simulink model "EngBrk_VNTP"  (R2016b)
settings: configuration reference "CodeGenConfigSet" (kept outside this file)
values from neighbouring files (symbols this model uses):
  COETS_EBSTATE_BRAKED = uint16(1)    [init_EngBrk_VNTP.m]
  ENGBRK_FIRED = uint8(0)    [init_EngBrk_VNTP.m]
  EngBrk_nEISGovOff_C = Calibration.Parameter    [init_EngBrk_VNTP.m]
  EngBrk_nEng_CUR = Calibration.Parameter    [init_EngBrk_VNTP.m]
  EngBrk_nEng_CURX = Calibration.Parameter    [init_EngBrk_VNTP.m]
  EngBrk_nEngThres_C = Calibration.Parameter    [init_EngBrk_VNTP.m]
  EngBrk_nOfsCA_CUR = Calibration.Parameter    [init_EngBrk_VNTP.m]
  EngBrk_nOfsCA_CURX = Calibration.Parameter    [init_EngBrk_VNTP.m]
  EngBrk_nOfsCADfct_C = Calibration.Parameter    [init_EngBrk_VNTP.m]
  EngBrk_rECRVlv_CUR = Calibration.Parameter    [init_EngBrk_VNTP.m]
  EngBrk_rECRVlv_CURX = Calibration.Parameter    [init_EngBrk_VNTP.m]
  EngBrk_rECRVlvHighDev_C = Calibration.Parameter    [init_EngBrk_VNTP.m]
  EngBrk_rECRVlvLowDev_C = Calibration.Parameter    [init_EngBrk_VNTP.m]
  EngBrk_rExhFlp_CUR = Calibration.Parameter    [init_EngBrk_VNTP.m]
  EngBrk_rExhFlp_CURX = Calibration.Parameter    [init_EngBrk_VNTP.m]
  EngBrk_rExhFlpHighDev_C = Calibration.Parameter    [init_EngBrk_VNTP.m]
  EngBrk_rExhFlpLowDev_C = Calibration.Parameter    [init_EngBrk_VNTP.m]
  EngBrk_rPT1TrqCurr_C = Calibration.Parameter    [init_EngBrk_VNTP.m]
  EngBrk_stDemMsk_C = Calibration.Parameter    [init_EngBrk_VNTP.m]
  EngBrk_swtECRVlv_C = Calibration.Parameter    [init_EngBrk_VNTP.m]
  EngBrk_swtExhFlp_C = Calibration.Parameter    [init_EngBrk_VNTP.m]
  EngBrk_tiDelayExhOff_C = Calibration.Parameter    [init_EngBrk_VNTP.m]
  EngBrk_tiPT1TrqCurr_C = Calibration.Parameter    [init_EngBrk_VNTP.m]
  EngBrk_tiRmp_C = Calibration.Parameter    [init_EngBrk_VNTP.m]
  EngBrk_tiRmpBlowOff_C = Calibration.Parameter    [init_EngBrk_VNTP.m]
  EngBrk_trqDeltaEnabECRVlv_GCUR = Calibration.Parameter    [init_EngBrk_VNTP.m]
  EngBrk_trqDeltaEnabECRVlv_GCURX = Calibration.Parameter    [init_EngBrk_VNTP.m]
  EngBrk_trqDeltaEnabExh_GCUR = Calibration.Parameter    [init_EngBrk_VNTP.m]
  EngBrk_trqDeltaEnabExh_GCURX = Calibration.Parameter    [init_EngBrk_VNTP.m]
  EngBrk_trqLimEnabECRVlv_GCUR = Calibration.Parameter    [init_EngBrk_VNTP.m]
  EngBrk_trqLimEnabECRVlv_GCURX = Calibration.Parameter    [init_EngBrk_VNTP.m]
  EngBrk_trqLimEnabExh_GCUR = Calibration.Parameter    [init_EngBrk_VNTP.m]
  EngBrk_trqLimEnabExh_GCURX = Calibration.Parameter    [init_EngBrk_VNTP.m]
  EngBrk_trqMax_GCUR = Calibration.Parameter    [init_EngBrk_VNTP.m]
  EngBrk_trqMax_GCURX = Calibration.Parameter    [init_EngBrk_VNTP.m]
  EngBrk_trqMaxDfct1_GCUR = Calibration.Parameter    [init_EngBrk_VNTP.m]
  EngBrk_trqMaxDfct1_GCURX = Calibration.Parameter    [init_EngBrk_VNTP.m]
  EngBrk_trqMaxDfct2_GCUR = Calibration.Parameter    [init_EngBrk_VNTP.m]
  EngBrk_trqMaxDfct2_GCURX = Calibration.Parameter    [init_EngBrk_VNTP.m]
  EngBrk_trqMaxDfct3_GCUR = Calibration.Parameter    [init_EngBrk_VNTP.m]
  EngBrk_trqMaxDfct3_GCURX = Calibration.Parameter    [init_EngBrk_VNTP.m]
  PRC_100 = uint8(0)    [init_EngBrk_VNTP.m]
  TRQ_MIN = int16(-3276)    [init_EngBrk_VNTP.m]
undefined symbols (not defined in the file or in its folder): EngBrk_VNTP_DT, HPUn_etaPmp_MAPY, Switch_conv
libraries: simulink x17, CXLib x10
settings Model: Creator=lenovo  LastModifiedBy=wangrui
settings ConfigSetRef: SourceLocation=Base Workspace

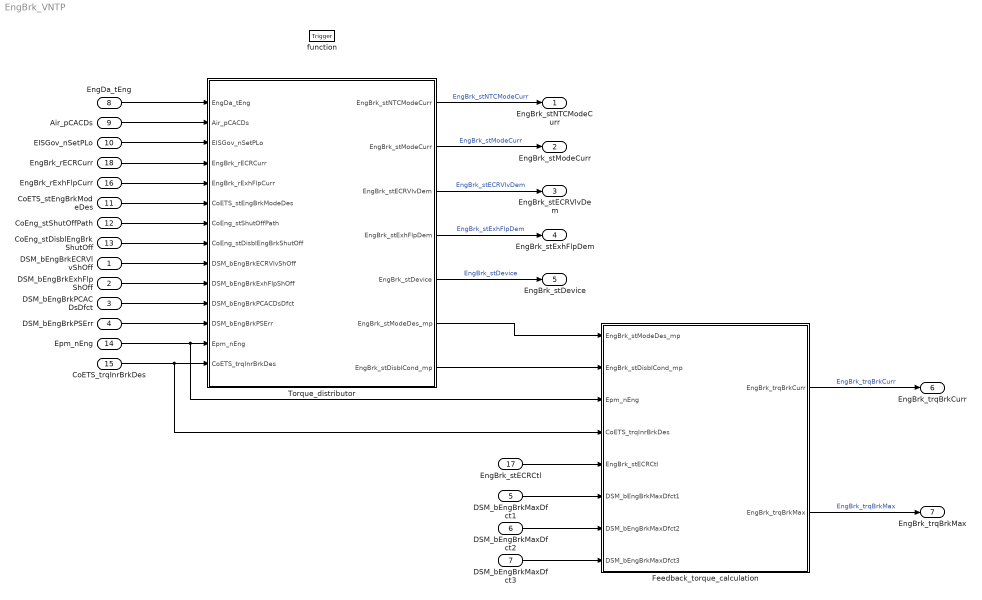
== system EngBrk_VNTP ==
  DSM_bEngBrkECRVlvShOff : Inport  Description=state of FId_EngBrkECRVlvShOff  OutMin=0  OutMax=1  OutDataTypeStr=boolean
  DSM_bEngBrkExhFlpShOff : Inport  Description=state of FId_EngBrkExhFlpShOff  Port=2  OutMin=0  OutMax=1  OutDataTypeStr=boolean
  DSM_bEngBrkPCACDsDfct : Inport  Description=state of FId_EngBrkPCACDsDfct  Port=3  OutMin=0  OutMax=1  OutDataTypeStr=boolean
  DSM_bEngBrkPSErr : Inport  Description=state of FId_EngBrkPSErr  Port=4  OutMin=0  OutMax=1  OutDataTypeStr=boolean
  DSM_bEngBrkMaxDfct1 : Inport  Description=state of FId_EngBrkMaxDfct1  Port=5  OutMin=0  OutMax=1  OutDataTypeStr=boolean
  DSM_bEngBrkMaxDfct2 : Inport  Description=state of FId_EngBrkMaxDfct2  Port=6  OutMin=0  OutMax=1  OutDataTypeStr=boolean
  DSM_bEngBrkMaxDfct3 : Inport  Description=state of FId_EngBrkMaxDfct3  Port=7  OutMin=0  OutMax=1  OutDataTypeStr=boolean
  EngDa_tEng : Inport  Tag=deg  Description=Engine temperature  Port=8  OutMin=-1000  OutMax=1000  OutDataTypeStr=Temp_deg
  Air_pCACDs : Inport  Tag=kPa  Description=Air pressure downstream of the charge air cooler  Port=9  OutMin=-3276.8  OutMax=3276.7  OutDataTypeStr=AirPressure_kPa
  EISGov_nSetPLo : Inport  Tag=rpm  Description=Lower limit of the speed interval (set point speed) of the EISGov  Port=10  OutMin=-12000  OutMax=12000  OutDataTypeStr=EngSpeed_rpm
  CoETS_stEngBrkModeDes : Inport  Description=Desired mode to VNTP  Port=11  OutMin=0  OutMax=65535  OutDataTypeStr=State_uint16
  CoEng_stShutOffPath : Inport  Description=Active shut-off paths resulting from active reversible,irreversible and afterrun shut-off paths  Port=12  OutMin=0  OutMax=65535  OutDataTypeStr=State_uint16
  CoEng_stDisblEngBrkShutOff : Inport  Description=|  Port=13  OutMin=0  OutMax=1  OutDataTypeStr=boolean
      | Status if injections are enabled although engine
      | brake can be active
  Epm_nEng : Inport  Tag=rpm  Description=Engine speed  Port=14  OutMin=0  OutMax=6000  OutDataTypeStr=EngSpeed_rpm
  CoETS_trqInrBrkDes : Inport  Tag=Nm  Description=Desired torque to VNTP Nm  Port=15  OutMin=-3276.8  OutMax=3276.7  OutDataTypeStr=Trq_Nm
  EngBrk_rExhFlpCurr : Inport  Tag=%  Description=Actual status (process signal) of exhaust flap  Port=16  OutMin=-200  OutMax=200  OutDataTypeStr=DutyCycle_rate
  EngBrk_stECRCtl : Inport  Description=Current status of the Engine compression release Valve(ECRVlv)  Port=17  OutMin=0  OutMax=255  OutDataTypeStr=State_uint8
  EngBrk_rECRCurr : Inport  Tag=%  Description=Current status of the Engine compression release Valve(ECRVlv) state machine  Port=18  OutMin=-200  OutMax=200  OutDataTypeStr=DutyCycle_rate
  function : TriggerPort  TriggerType=function-call  VariantControl=Variant
  Feedback_torque_calculation : Subsystem
  Torque_distributor : Subsystem
  EngBrk_stNTCModeCurr : Outport  Description=VNTP status for NTC, TRUE if active (CRER or ExhFlp)  OutMin=0  OutMax=255  OutDataTypeStr=State_uint8
  EngBrk_stModeCurr : Outport  Description=VNTP status, TRUE if active (CRER or ExhFlp and injection shut-off)  Port=2  OutMin=0  OutMax=255  OutDataTypeStr=State_uint8
  EngBrk_stECRVlvDem : Outport  Description=Activation demand to Engine compression release Valve(ECRVlv)  Port=3  OutMin=0  OutMax=255  OutDataTypeStr=State_uint8
  EngBrk_stExhFlpDem : Outport  Description=Activation demand to exhaust flap  Port=4  OutMin=0  OutMax=1  OutDataTypeStr=boolean
  EngBrk_stDevice : Outport  Description=Device actuated by VNTP, used as map selection for ratio and pressure setpoint calculation  Port=5  OutMin=0  OutMax=255  OutDataTypeStr=State_uint8
  EngBrk_trqBrkCurr : Outport  Tag=Nm  Description=Current engine brake torque  Port=6  OutMin=-3276.8  OutMax=3276.7  OutDataTypeStr=Trq_Nm
  EngBrk_trqBrkMax : Outport  Tag=Nm  Description=Maximum available engine brake torque  Port=7  OutMin=-3276.8  OutMax=3276.7  OutDataTypeStr=Trq_Nm
  wires:
  EngBrk_rECRCurr/1 -> Torque_distributor/4(EngBrk_rECRCurr)
  Epm_nEng/1 -> Feedback_torque_calculation/3(Epm_nEng), Torque_distributor/13(Epm_nEng)
  Torque_distributor/4(EngBrk_stExhFlpDem) -> EngBrk_stExhFlpDem/1  "EngBrk_stExhFlpDem"
  EISGov_nSetPLo/1 -> Torque_distributor/3(EISGov_nSetPLo)
  CoETS_trqInrBrkDes/1 -> Feedback_torque_calculation/4(CoETS_trqInrBrkDes), Torque_distributor/14(CoETS_trqInrBrkDes)
  CoEng_stDisblEngBrkShutOff/1 -> Torque_distributor/8(CoEng_stDisblEngBrkShutOff)
  Air_pCACDs/1 -> Torque_distributor/2(Air_pCACDs)
  Torque_distributor/2(EngBrk_stModeCurr) -> EngBrk_stModeCurr/1  "EngBrk_stModeCurr"
  Torque_distributor/7(EngBrk_stDisblCond_mp) -> Feedback_torque_calculation/2(EngBrk_stDisblCond_mp)
  Torque_distributor/3(EngBrk_stECRVlvDem) -> EngBrk_stECRVlvDem/1  "EngBrk_stECRVlvDem"
  Feedback_torque_calculation/2(EngBrk_trqBrkMax) -> EngBrk_trqBrkMax/1  "EngBrk_trqBrkMax"
  Feedback_torque_calculation/1(EngBrk_trqBrkCurr) -> EngBrk_trqBrkCurr/1  "EngBrk_trqBrkCurr"
  Torque_distributor/5(EngBrk_stDevice) -> EngBrk_stDevice/1  "EngBrk_stDevice"
  CoETS_stEngBrkModeDes/1 -> Torque_distributor/6(CoETS_stEngBrkModeDes)
  EngBrk_stECRCtl/1 -> Feedback_torque_calculation/5(EngBrk_stECRCtl)
  CoEng_stShutOffPath/1 -> Torque_distributor/7(CoEng_stShutOffPath)
  Torque_distributor/6(EngBrk_stModeDes_mp) -> Feedback_torque_calculation/1(EngBrk_stModeDes_mp)
  EngDa_tEng/1 -> Torque_distributor/1(EngDa_tEng)
  EngBrk_rExhFlpCurr/1 -> Torque_distributor/5(EngBrk_rExhFlpCurr)
  Torque_distributor/1(EngBrk_stNTCModeCurr) -> EngBrk_stNTCModeCurr/1  "EngBrk_stNTCModeCurr"
  DSM_bEngBrkMaxDfct1/1 -> Feedback_torque_calculation/6(DSM_bEngBrkMaxDfct1)
  DSM_bEngBrkMaxDfct2/1 -> Feedback_torque_calculation/7(DSM_bEngBrkMaxDfct2)
  DSM_bEngBrkMaxDfct3/1 -> Feedback_torque_calculation/8(DSM_bEngBrkMaxDfct3)
  DSM_bEngBrkECRVlvShOff/1 -> Torque_distributor/9(DSM_bEngBrkECRVlvShOff)
  DSM_bEngBrkExhFlpShOff/1 -> Torque_distributor/10(DSM_bEngBrkExhFlpShOff)
  DSM_bEngBrkPCACDsDfct/1 -> Torque_distributor/11(DSM_bEngBrkPCACDsDfct)
  DSM_bEngBrkPSErr/1 -> Torque_distributor/12(DSM_bEngBrkPSErr)

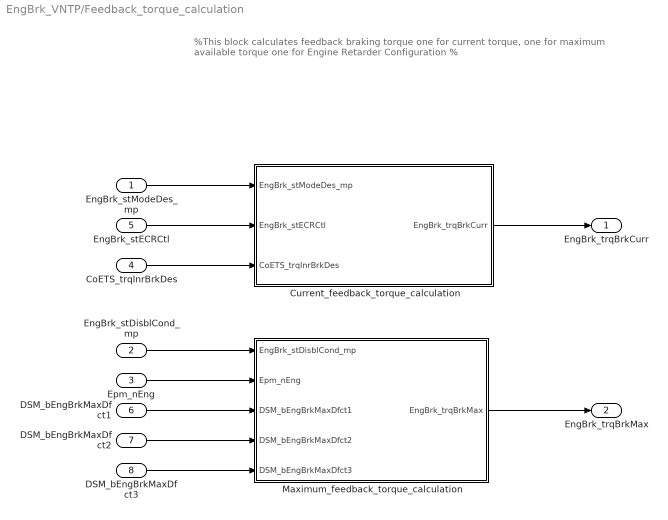
== system EngBrk_VNTP/Feedback_torque_calculation ==
  note: %This block calculates feedback braking torque
      | one for current torque,
      | one for maximum available torque
      | one for Engine Retarder Configuration %
  EngBrk_stModeDes_mp : Inport
  EngBrk_stDisblCond_mp : Inport  Port=2
  Epm_nEng : Inport  Port=3
  CoETS_trqInrBrkDes : Inport  Port=4
  EngBrk_stECRCtl : Inport  Port=5
  DSM_bEngBrkMaxDfct1 : Inport  Description=state of FId_EngBrkMaxDfct1  Port=6  OutMin=0  OutMax=1  OutDataTypeStr=boolean
  DSM_bEngBrkMaxDfct2 : Inport  Description=state of FId_EngBrkMaxDfct2  Port=7  OutMin=0  OutMax=1  OutDataTypeStr=boolean
  DSM_bEngBrkMaxDfct3 : Inport  Description=state of FId_EngBrkMaxDfct3  Port=8  OutMin=0  OutMax=1  OutDataTypeStr=boolean
  Current_feedback_torque_calculation : Subsystem
  Maximum_feedback_torque_calculation : Subsystem
  EngBrk_trqBrkCurr : Outport
  EngBrk_trqBrkMax : Outport  Port=2
  wires:
  Maximum_feedback_torque_calculation/1(EngBrk_trqBrkMax) -> EngBrk_trqBrkMax/1
  Current_feedback_torque_calculation/1(EngBrk_trqBrkCurr) -> EngBrk_trqBrkCurr/1
  Epm_nEng/1 -> Maximum_feedback_torque_calculation/2(Epm_nEng)
  EngBrk_stDisblCond_mp/1 -> Maximum_feedback_torque_calculation/1(EngBrk_stDisblCond_mp)
  CoETS_trqInrBrkDes/1 -> Current_feedback_torque_calculation/3(CoETS_trqInrBrkDes)
  EngBrk_stECRCtl/1 -> Current_feedback_torque_calculation/2(EngBrk_stECRCtl)
  EngBrk_stModeDes_mp/1 -> Current_feedback_torque_calculation/1(EngBrk_stModeDes_mp)
  DSM_bEngBrkMaxDfct1/1 -> Maximum_feedback_torque_calculation/3(DSM_bEngBrkMaxDfct1)
  DSM_bEngBrkMaxDfct2/1 -> Maximum_feedback_torque_calculation/4(DSM_bEngBrkMaxDfct2)
  DSM_bEngBrkMaxDfct3/1 -> Maximum_feedback_torque_calculation/5(DSM_bEngBrkMaxDfct3)

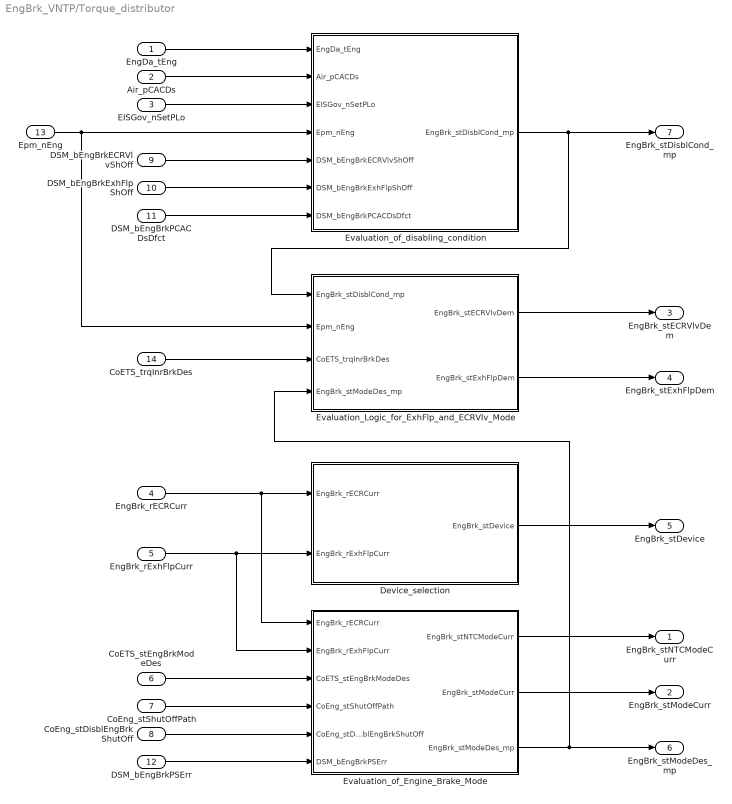
== system EngBrk_VNTP/Torque_distributor ==
  EngDa_tEng : Inport
  Air_pCACDs : Inport  Port=2
  EISGov_nSetPLo : Inport  Port=3
  EngBrk_rECRCurr : Inport  Port=4
  EngBrk_rExhFlpCurr : Inport  Port=5
  CoETS_stEngBrkModeDes : Inport  Port=6
  CoEng_stShutOffPath : Inport  Port=7
  CoEng_stDisblEngBrkShutOff : Inport  Port=8
  DSM_bEngBrkECRVlvShOff : Inport  Description=state of FId_EngBrkECRVlvShOff  Port=9  OutMin=0  OutMax=1  OutDataTypeStr=boolean
  DSM_bEngBrkExhFlpShOff : Inport  Description=state of FId_EngBrkExhFlpShOff  Port=10  OutMin=0  OutMax=1  OutDataTypeStr=boolean
  DSM_bEngBrkPCACDsDfct : Inport  Description=state of FId_EngBrkPCACDsDfct  Port=11  OutMin=0  OutMax=1  OutDataTypeStr=boolean
  DSM_bEngBrkPSErr : Inport  Description=state of FId_EngBrkPSErr  Port=12  OutMin=0  OutMax=1  OutDataTypeStr=boolean
  Epm_nEng : Inport  Port=13
  CoETS_trqInrBrkDes : Inport  Port=14
  Device_selection : Subsystem
  Evaluation_Logic_for_ExhFlp_and_ECRVlv_Mode : Subsystem
  Evaluation_of_Engine_Brake_Mode : Subsystem
  Evaluation_of_disabling_condition : Subsystem
  EngBrk_stNTCModeCurr : Outport
  EngBrk_stModeCurr : Outport  Port=2
  EngBrk_stECRVlvDem : Outport  Port=3
  EngBrk_stExhFlpDem : Outport  Port=4
  EngBrk_stDevice : Outport  Port=5
  EngBrk_stModeDes_mp : Outport  Port=6
  EngBrk_stDisblCond_mp : Outport  Port=7
  wires:
  Device_selection/1(EngBrk_stDevice) -> EngBrk_stDevice/1
  Evaluation_Logic_for_ExhFlp_and_ECRVlv_Mode/2(EngBrk_stExhFlpDem) -> EngBrk_stExhFlpDem/1
  Evaluation_Logic_for_ExhFlp_and_ECRVlv_Mode/1(EngBrk_stECRVlvDem) -> EngBrk_stECRVlvDem/1
  Evaluation_of_Engine_Brake_Mode/2(EngBrk_stModeCurr) -> EngBrk_stModeCurr/1
  Evaluation_of_Engine_Brake_Mode/1(EngBrk_stNTCModeCurr) -> EngBrk_stNTCModeCurr/1
  CoETS_trqInrBrkDes/1 -> Evaluation_Logic_for_ExhFlp_and_ECRVlv_Mode/3(CoETS_trqInrBrkDes)
  Epm_nEng/1 -> Evaluation_of_disabling_condition/4(Epm_nEng), Evaluation_Logic_for_ExhFlp_and_ECRVlv_Mode/2(Epm_nEng)
  Evaluation_of_Engine_Brake_Mode/3(EngBrk_stModeDes_mp) -> EngBrk_stModeDes_mp/1, Evaluation_Logic_for_ExhFlp_and_ECRVlv_Mode/4(EngBrk_stModeDes_mp)
  CoEng_stDisblEngBrkShutOff/1 -> Evaluation_of_Engine_Brake_Mode/5(CoEng_stDisblEngBrkShutOff)
  CoEng_stShutOffPath/1 -> Evaluation_of_Engine_Brake_Mode/4(CoEng_stShutOffPath)
  CoETS_stEngBrkModeDes/1 -> Evaluation_of_Engine_Brake_Mode/3(CoETS_stEngBrkModeDes)
  EngBrk_rExhFlpCurr/1 -> Evaluation_of_Engine_Brake_Mode/2(EngBrk_rExhFlpCurr), Device_selection/2(EngBrk_rExhFlpCurr)
  EngBrk_rECRCurr/1 -> Device_selection/1(EngBrk_rECRCurr), Evaluation_of_Engine_Brake_Mode/1(EngBrk_rECRCurr)
  Evaluation_of_disabling_condition/1(EngBrk_stDisblCond_mp) -> EngBrk_stDisblCond_mp/1, Evaluation_Logic_for_ExhFlp_and_ECRVlv_Mode/1(EngBrk_stDisblCond_mp)
  EISGov_nSetPLo/1 -> Evaluation_of_disabling_condition/3(EISGov_nSetPLo)
  Air_pCACDs/1 -> Evaluation_of_disabling_condition/2(Air_pCACDs)
  EngDa_tEng/1 -> Evaluation_of_disabling_condition/1(EngDa_tEng)
  DSM_bEngBrkECRVlvShOff/1 -> Evaluation_of_disabling_condition/5(DSM_bEngBrkECRVlvShOff)
  DSM_bEngBrkExhFlpShOff/1 -> Evaluation_of_disabling_condition/6(DSM_bEngBrkExhFlpShOff)
  DSM_bEngBrkPCACDsDfct/1 -> Evaluation_of_disabling_condition/7(DSM_bEngBrkPCACDsDfct)
  DSM_bEngBrkPSErr/1 -> Evaluation_of_Engine_Brake_Mode/6(DSM_bEngBrkPSErr)

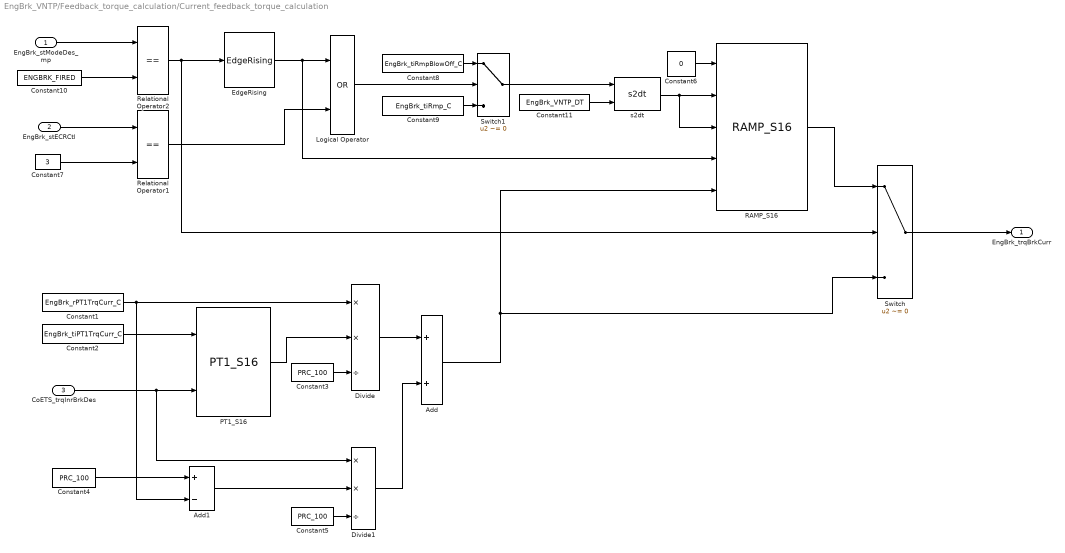
== system EngBrk_VNTP/Feedback_torque_calculation/Current_feedback_torque_calculation ==
  EngBrk_stModeDes_mp : Inport
  EngBrk_stECRCtl : Inport  Port=2
  CoETS_trqInrBrkDes : Inport  Port=3
  Add : Sum  SaturateOnIntegerOverflow=on  InputSameDT=on
  Add1 : Sum  Inputs=+-  OutDataTypeStr=Inherit: Inherit via back propagation  SaturateOnIntegerOverflow=on  InputSameDT=on
  Constant1 : Constant  Value=EngBrk_rPT1TrqCurr_C
  Constant10 : Constant  Value=ENGBRK_FIRED  OutDataTypeStr=Inherit: Inherit via back propagation
  Constant11 : Constant  Value=EngBrk_VNTP_DT  OutDataTypeStr=Inherit: Inherit via back propagation
  Constant2 : Constant  Value=EngBrk_tiPT1TrqCurr_C
  Constant3 : Constant  Value=PRC_100  OutDataTypeStr=DutyCycle_rate
  Constant4 : Constant  Value=PRC_100  OutDataTypeStr=Inherit: Inherit via back propagation
  Constant5 : Constant  Value=PRC_100  OutDataTypeStr=DutyCycle_rate
  Constant6 : Constant  Value=0  OutDataTypeStr=Inherit: Inherit via back propagation
  Constant7 : Constant  Value=3  OutDataTypeStr=Inherit: Inherit via back propagation
  Constant8 : Constant  Value=EngBrk_tiRmpBlowOff_C
  Constant9 : Constant  Value=EngBrk_tiRmp_C
  Divide : Product  Inputs=**/  OutDataTypeStr=Trq_Nm  SaturateOnIntegerOverflow=on
  Divide1 : Product  Inputs=**/  OutDataTypeStr=Trq_Nm  SaturateOnIntegerOverflow=on
  EdgeRising : CXLib/EdgeRising
  Logical Operator : Logic  Operator=OR  OutDataTypeStr=boolean
  PT1_S16 : CXLib/PT1_S16  offset=0
  RAMP_S16 : CXLib/RAMP_S16
  Relational Operator1 : RelationalOperator  Operator===  OutDataTypeStr=boolean  RndMeth=Simplest  InputSameDT=on
  Relational Operator2 : RelationalOperator  Operator===  OutDataTypeStr=boolean  RndMeth=Simplest  InputSameDT=on
  Switch : Switch  Criteria=u2 ~= 0  SaturateOnIntegerOverflow=on  InputSameDT=on
  Switch1 : Switch  Criteria=u2 ~= 0  SaturateOnIntegerOverflow=on  InputSameDT=on
  s2dt : CXLib/s2dt
  EngBrk_trqBrkCurr : Outport
  wires:
  Constant11/1 -> s2dt/2
  Switch1/1 -> s2dt/1
  s2dt/1 -> RAMP_S16/2, RAMP_S16/3
  Relational Operator1/1 -> Logical Operator/2
  EdgeRising/1 -> Logical Operator/1, RAMP_S16/4
  Relational Operator2/1 -> Switch/2, EdgeRising/1
  Constant10/1 -> Relational Operator2/2
  EngBrk_stModeDes_mp/1 -> Relational Operator2/1
  Constant9/1 -> Switch1/3
  Constant8/1 -> Switch1/1
  Logical Operator/1 -> Switch1/2
  Constant7/1 -> Relational Operator1/2
  EngBrk_stECRCtl/1 -> Relational Operator1/1
  Constant6/1 -> RAMP_S16/1
  Switch/1 -> EngBrk_trqBrkCurr/1
  RAMP_S16/1 -> Switch/1
  Add/1 -> RAMP_S16/5, Switch/3
  Divide1/1 -> Add/2
  Constant5/1 -> Divide1/3
  Add1/1 -> Divide1/2
  Constant4/1 -> Add1/1
  Divide/1 -> Add/1
  Constant3/1 -> Divide/3
  Constant1/1 -> Add1/2, Divide/1
  PT1_S16/1 -> Divide/2
  CoETS_trqInrBrkDes/1 -> Divide1/1, PT1_S16/2
  Constant2/1 -> PT1_S16/1

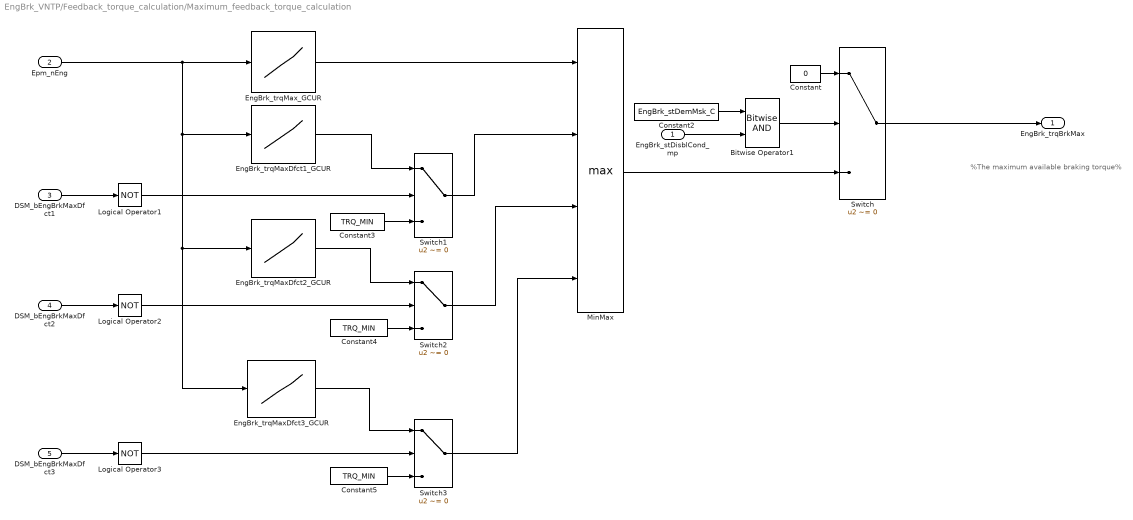
== system EngBrk_VNTP/Feedback_torque_calculation/Maximum_feedback_torque_calculation ==
  note: %The maximum available braking torque%
  EngBrk_stDisblCond_mp : Inport
  Epm_nEng : Inport  Port=2
  DSM_bEngBrkMaxDfct1 : Inport  Description=state of FId_EngBrkMaxDfct1  Port=3  OutMin=0  OutMax=1  OutDataTypeStr=boolean
  DSM_bEngBrkMaxDfct2 : Inport  Description=state of FId_EngBrkMaxDfct2  Port=4  OutMin=0  OutMax=1  OutDataTypeStr=boolean
  DSM_bEngBrkMaxDfct3 : Inport  Description=state of FId_EngBrkMaxDfct3  Port=5  OutMin=0  OutMax=1  OutDataTypeStr=boolean
  Bitwise Operator1 : simulink/Logic and Bit Operations/Bitwise Operator  logicop=AND  UseBitMask=off  NumInputPorts=2  BitMask=bin2dec('00000001')  BitMaskRealWorld=Stored Integer
  Constant : Constant  Value=0  OutDataTypeStr=Inherit: Inherit via back propagation
  Constant2 : Constant  Value=EngBrk_stDemMsk_C
  Constant3 : Constant  Value=TRQ_MIN  OutDataTypeStr=Trq_Nm
  Constant4 : Constant  Value=TRQ_MIN  OutDataTypeStr=Trq_Nm
  Constant5 : Constant  Value=TRQ_MIN  OutDataTypeStr=Trq_Nm
  EngBrk_trqMaxDfct1_GCUR : Lookup_n-D  NumberOfTableDimensions=1  BreakpointsForDimension1=EngBrk_trqMaxDfct1_GCURX  BreakpointsForDimension2=HPUn_etaPmp_MAPY  IndexSearchMethod=Linear search  BeginIndexSearchUsingPreviousIndexResult=on  Table=EngBrk_trqMaxDfct1_GCUR  ExtrapMethod=Clip  UseLastTableValue=on  InternalRulePriority=Speed  OutDataTypeStr=Inherit: Inherit via back propagation  SaturateOnIntegerOverflow=on
  EngBrk_trqMaxDfct2_GCUR : Lookup_n-D  NumberOfTableDimensions=1  BreakpointsForDimension1=EngBrk_trqMaxDfct2_GCURX  BreakpointsForDimension2=HPUn_etaPmp_MAPY  IndexSearchMethod=Linear search  BeginIndexSearchUsingPreviousIndexResult=on  Table=EngBrk_trqMaxDfct2_GCUR  ExtrapMethod=Clip  UseLastTableValue=on  InternalRulePriority=Speed  OutDataTypeStr=Inherit: Inherit via back propagation  SaturateOnIntegerOverflow=on
  EngBrk_trqMaxDfct3_GCUR : Lookup_n-D  NumberOfTableDimensions=1  BreakpointsForDimension1=EngBrk_trqMaxDfct3_GCURX  BreakpointsForDimension2=HPUn_etaPmp_MAPY  IndexSearchMethod=Linear search  BeginIndexSearchUsingPreviousIndexResult=on  Table=EngBrk_trqMaxDfct3_GCUR  ExtrapMethod=Clip  UseLastTableValue=on  InternalRulePriority=Speed  OutDataTypeStr=Inherit: Inherit via back propagation  SaturateOnIntegerOverflow=on
  EngBrk_trqMax_GCUR : Lookup_n-D  NumberOfTableDimensions=1  BreakpointsForDimension1=EngBrk_trqMax_GCURX  BreakpointsForDimension2=HPUn_etaPmp_MAPY  IndexSearchMethod=Linear search  BeginIndexSearchUsingPreviousIndexResult=on  Table=EngBrk_trqMax_GCUR  ExtrapMethod=Clip  UseLastTableValue=on  InternalRulePriority=Speed  OutDataTypeStr=Inherit: Inherit via back propagation  SaturateOnIntegerOverflow=on
  Logical Operator1 : Logic  Operator=NOT  AllPortsSameDT=off  OutDataTypeStr=boolean
  Logical Operator2 : Logic  Operator=NOT  AllPortsSameDT=off  OutDataTypeStr=boolean
  Logical Operator3 : Logic  Operator=NOT  AllPortsSameDT=off  OutDataTypeStr=boolean
  MinMax : MinMax  Function=max  Inputs=4  SaturateOnIntegerOverflow=on  InputSameDT=on
  Switch{,1..3} (4 alike) : Switch  Criteria=u2 ~= 0  SaturateOnIntegerOverflow=on  InputSameDT=on
  EngBrk_trqBrkMax : Outport
  wires:
  Switch/1 -> EngBrk_trqBrkMax/1
  Bitwise Operator1/1 -> Switch/2
  Constant/1 -> Switch/1
  MinMax/1 -> Switch/3
  Switch3/1 -> MinMax/4
  Switch2/1 -> MinMax/3
  Switch1/1 -> MinMax/2
  Logical Operator1/1 -> Switch1/2
  Logical Operator3/1 -> Switch3/2
  Logical Operator2/1 -> Switch2/2
  DSM_bEngBrkMaxDfct3/1 -> Logical Operator3/1
  DSM_bEngBrkMaxDfct2/1 -> Logical Operator2/1
  DSM_bEngBrkMaxDfct1/1 -> Logical Operator1/1
  Constant5/1 -> Switch3/3
  Constant4/1 -> Switch2/3
  Constant3/1 -> Switch1/3
  EngBrk_trqMaxDfct3_GCUR/1 -> Switch3/1
  EngBrk_trqMaxDfct2_GCUR/1 -> Switch2/1
  EngBrk_trqMaxDfct1_GCUR/1 -> Switch1/1
  EngBrk_trqMax_GCUR/1 -> MinMax/1
  Epm_nEng/1 -> EngBrk_trqMax_GCUR/1, EngBrk_trqMaxDfct1_GCUR/1, EngBrk_trqMaxDfct2_GCUR/1, EngBrk_trqMaxDfct3_GCUR/1
  Constant2/1 -> Bitwise Operator1/1
  EngBrk_stDisblCond_mp/1 -> Bitwise Operator1/2

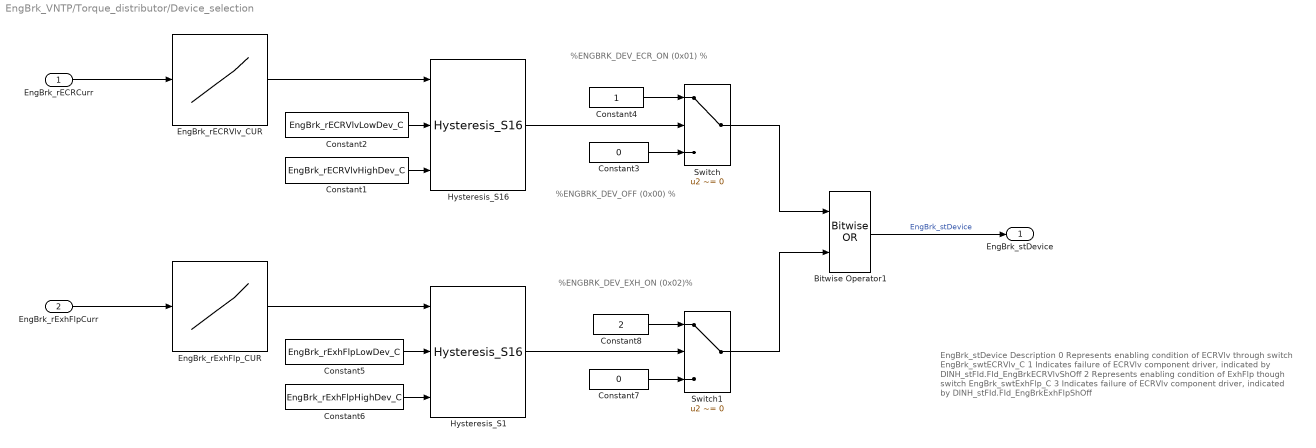
== system EngBrk_VNTP/Torque_distributor/Device_selection ==
  note: EngBrk_stDevice
      | Description
      |
      | 0
      | Represents enabling condition of ECRVlv through switch EngBrk_swtECRVlv_C
      |
      | 1
      | Indicates failure of ECRVlv component driver, indicated by DINH_stFId.FId_EngBrkECRVlvShOff
      |
      | 2
      | Represents enabling condition of ExhFlp though switch EngBrk_swtExhFlp_C
      |
      | 3
      | Indicates failure of ECRVlv component driver, indicated by DINH_stFId.FId_EngBrkExhFlpShOff
  note: %ENGBRK_DEV_OFF (0x00) %
  note: %ENGBRK_DEV_ECR_ON (0x01) %
  note: %ENGBRK_DEV_EXH_ON (0x02)%
  EngBrk_rECRCurr : Inport
  EngBrk_rExhFlpCurr : Inport  Port=2
  Bitwise Operator1 : simulink/Logic and Bit Operations/Bitwise Operator  logicop=OR  UseBitMask=off  NumInputPorts=2  BitMask=bin2dec('00000001')  BitMaskRealWorld=Stored Integer
  Constant1 : Constant  Value=EngBrk_rECRVlvHighDev_C
  Constant2 : Constant  Value=EngBrk_rECRVlvLowDev_C
  Constant3 : Constant  Value=0  OutDataTypeStr=Inherit: Inherit via back propagation
  Constant4 : Constant  OutDataTypeStr=Inherit: Inherit via back propagation
  Constant5 : Constant  Value=EngBrk_rExhFlpLowDev_C
  Constant6 : Constant  Value=EngBrk_rExhFlpHighDev_C
  Constant7 : Constant  Value=0  OutDataTypeStr=Inherit: Inherit via back propagation
  Constant8 : Constant  Value=2  OutDataTypeStr=Inherit: Inherit via back propagation
  EngBrk_rECRVlv_CUR : Lookup_n-D  NumberOfTableDimensions=1  BreakpointsForDimension1=EngBrk_rECRVlv_CURX  BreakpointsForDimension2=HPUn_etaPmp_MAPY  IndexSearchMethod=Linear search  BeginIndexSearchUsingPreviousIndexResult=on  Table=EngBrk_rECRVlv_CUR  ExtrapMethod=Clip  UseLastTableValue=on  InternalRulePriority=Speed  OutDataTypeStr=Inherit: Inherit via back propagation  SaturateOnIntegerOverflow=on
  EngBrk_rExhFlp_CUR : Lookup_n-D  NumberOfTableDimensions=1  BreakpointsForDimension1=EngBrk_rExhFlp_CURX  BreakpointsForDimension2=HPUn_etaPmp_MAPY  IndexSearchMethod=Linear search  BeginIndexSearchUsingPreviousIndexResult=on  Table=EngBrk_rExhFlp_CUR  ExtrapMethod=Clip  UseLastTableValue=on  InternalRulePriority=Speed  OutDataTypeStr=Inherit: Inherit via back propagation  SaturateOnIntegerOverflow=on
  Hysteresis_S1 : CXLib/Hysteresis_S16
  Hysteresis_S16 : CXLib/Hysteresis_S16
  Switch : Switch  Criteria=u2 ~= 0  SaturateOnIntegerOverflow=on  InputSameDT=on
  Switch1 : Switch  Criteria=u2 ~= 0  SaturateOnIntegerOverflow=on  InputSameDT=on
  EngBrk_stDevice : Outport
  wires:
  Bitwise Operator1/1 -> EngBrk_stDevice/1  "EngBrk_stDevice"
  Switch1/1 -> Bitwise Operator1/2
  Switch/1 -> Bitwise Operator1/1
  Constant8/1 -> Switch1/1
  Constant7/1 -> Switch1/3
  Hysteresis_S1/1 -> Switch1/2
  Constant6/1 -> Hysteresis_S1/3
  Constant5/1 -> Hysteresis_S1/2
  EngBrk_rExhFlp_CUR/1 -> Hysteresis_S1/1
  EngBrk_rExhFlpCurr/1 -> EngBrk_rExhFlp_CUR/1
  Constant4/1 -> Switch/1
  Constant3/1 -> Switch/3
  Hysteresis_S16/1 -> Switch/2
  Constant1/1 -> Hysteresis_S16/3
  Constant2/1 -> Hysteresis_S16/2
  EngBrk_rECRVlv_CUR/1 -> Hysteresis_S16/1
  EngBrk_rECRCurr/1 -> EngBrk_rECRVlv_CUR/1

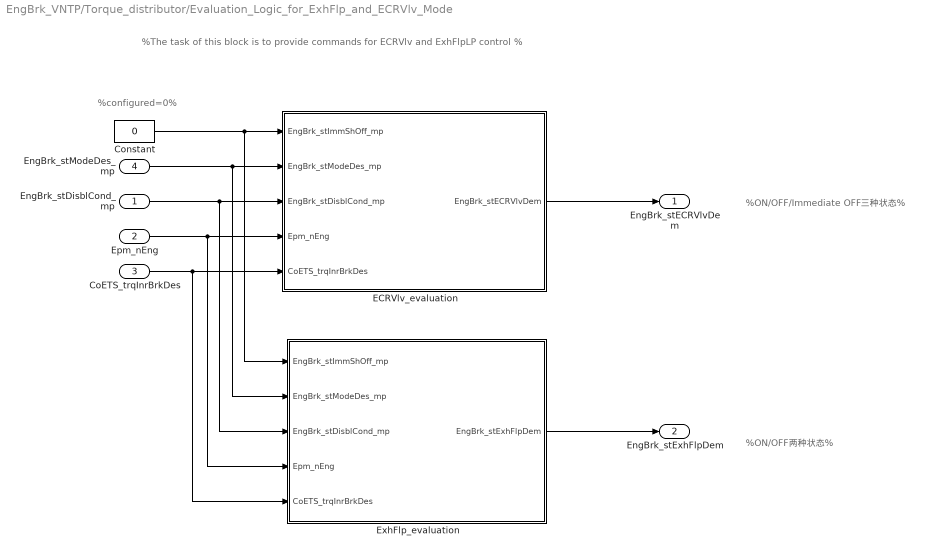
== system EngBrk_VNTP/Torque_distributor/Evaluation_Logic_for_ExhFlp_and_ECRVlv_Mode ==
  note: %ON/OFF/Immediate OFF三种状态%
  note: %The task of this block is to provide commands for ECRVlv and ExhFlpLP control %
  note: %ON/OFF两种状态%
  note: %configured=0%
  EngBrk_stDisblCond_mp : Inport
  Epm_nEng : Inport  Port=2
  CoETS_trqInrBrkDes : Inport  Port=3
  EngBrk_stModeDes_mp : Inport  Port=4
  Constant : Constant  Value=0  OutDataTypeStr=boolean
  ECRVlv_evaluation : Subsystem
  ExhFlp_evaluation : Subsystem
  EngBrk_stECRVlvDem : Outport
  EngBrk_stExhFlpDem : Outport  Port=2
  wires:
  ExhFlp_evaluation/1(EngBrk_stExhFlpDem) -> EngBrk_stExhFlpDem/1
  ECRVlv_evaluation/1(EngBrk_stECRVlvDem) -> EngBrk_stECRVlvDem/1
  CoETS_trqInrBrkDes/1 -> ECRVlv_evaluation/5(CoETS_trqInrBrkDes), ExhFlp_evaluation/5(CoETS_trqInrBrkDes)
  Epm_nEng/1 -> ECRVlv_evaluation/4(Epm_nEng), ExhFlp_evaluation/4(Epm_nEng)
  EngBrk_stDisblCond_mp/1 -> ECRVlv_evaluation/3(EngBrk_stDisblCond_mp), ExhFlp_evaluation/3(EngBrk_stDisblCond_mp)
  EngBrk_stModeDes_mp/1 -> ECRVlv_evaluation/2(EngBrk_stModeDes_mp), ExhFlp_evaluation/2(EngBrk_stModeDes_mp)
  Constant/1 -> ECRVlv_evaluation/1(EngBrk_stImmShOff_mp), ExhFlp_evaluation/1(EngBrk_stImmShOff_mp)

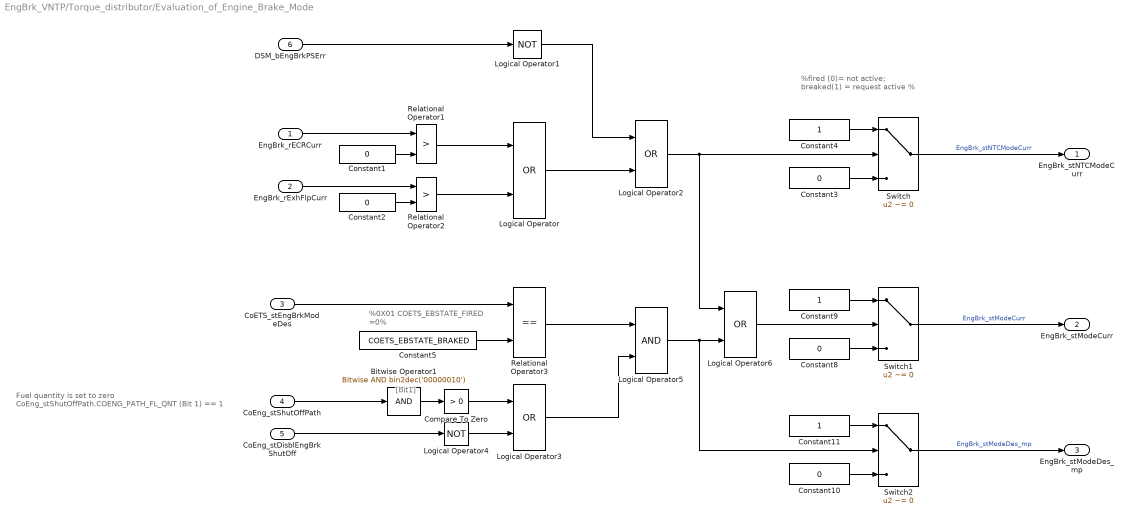
== system EngBrk_VNTP/Torque_distributor/Evaluation_of_Engine_Brake_Mode ==
  note: %fired (0)= not active;
      | breaked(1) = request active %
  note: Fuel quantity is set to zero
      | CoEng_stShutOffPath.COENG_PATH_FL_QNT (Bit 1) == 1
  note: [bit1]
  note: %0X01
      | COETS_EBSTATE_FIRED =0%
  EngBrk_rECRCurr : Inport
  EngBrk_rExhFlpCurr : Inport  Port=2
  CoETS_stEngBrkModeDes : Inport  Port=3
  CoEng_stShutOffPath : Inport  Port=4
  CoEng_stDisblEngBrkShutOff : Inport  Port=5
  DSM_bEngBrkPSErr : Inport  Description=state of FId_EngBrkPSErr  Port=6  OutMin=0  OutMax=1  OutDataTypeStr=boolean
  Bitwise Operator1 : simulink/Logic and Bit Operations/Bitwise Operator  logicop=AND  UseBitMask=on  BitMask=bin2dec('00000010')  BitMaskRealWorld=Stored Integer
  Compare To Zero : simulink/Logic and Bit Operations/Compare To Zero  relop=>  OutDataTypeStr=boolean
  Constant{1..3,8,10} (5 alike) : Constant  Value=0  OutDataTypeStr=Inherit: Inherit via back propagation
  Constant11 : Constant  OutDataTypeStr=Inherit: Inherit via back propagation
  Constant4 : Constant  OutDataTypeStr=Inherit: Inherit via back propagation
  Constant5 : Constant  Value=COETS_EBSTATE_BRAKED  OutDataTypeStr=State_uint16
  Constant9 : Constant  OutDataTypeStr=Inherit: Inherit via back propagation
  Logical Operator{,2..3,6} (4 alike) : Logic  Operator=OR  OutDataTypeStr=boolean
  Logical Operator1 : Logic  Operator=NOT  AllPortsSameDT=off  OutDataTypeStr=boolean
  Logical Operator4 : Logic  Operator=NOT  AllPortsSameDT=off  OutDataTypeStr=boolean
  Logical Operator5 : Logic  OutDataTypeStr=boolean
  Relational Operator1 : RelationalOperator  Operator=>  OutDataTypeStr=boolean  RndMeth=Simplest  InputSameDT=on
  Relational Operator2 : RelationalOperator  Operator=>  OutDataTypeStr=boolean  RndMeth=Simplest  InputSameDT=on
  Relational Operator3 : RelationalOperator  Operator===  OutDataTypeStr=boolean  RndMeth=Simplest  InputSameDT=on
  Switch : Switch  Criteria=u2 ~= 0  SaturateOnIntegerOverflow=on  InputSameDT=on
  Switch1 : Switch  Criteria=u2 ~= 0  SaturateOnIntegerOverflow=on  InputSameDT=on
  Switch2 : Switch  Criteria=u2 ~= 0  SaturateOnIntegerOverflow=on  InputSameDT=on
  EngBrk_stNTCModeCurr : Outport
  EngBrk_stModeCurr : Outport  Port=2
  EngBrk_stModeDes_mp : Outport  Port=3
  wires:
  Constant11/1 -> Switch2/1
  Constant10/1 -> Switch2/3
  Logical Operator5/1 -> Logical Operator6/2, Switch2/2
  Constant9/1 -> Switch1/1
  Constant8/1 -> Switch1/3
  Logical Operator6/1 -> Switch1/2
  Constant1/1 -> Relational Operator1/2
  Switch2/1 -> EngBrk_stModeDes_mp/1  "EngBrk_stModeDes_mp"
  Switch1/1 -> EngBrk_stModeCurr/1  "EngBrk_stModeCurr"
  Relational Operator3/1 -> Logical Operator5/1
  Logical Operator3/1 -> Logical Operator5/2
  Logical Operator4/1 -> Logical Operator3/2
  CoEng_stDisblEngBrkShutOff/1 -> Logical Operator4/1
  Compare To Zero/1 -> Logical Operator3/1
  Bitwise Operator1/1 -> Compare To Zero/1
  Constant5/1 -> Relational Operator3/2
  CoETS_stEngBrkModeDes/1 -> Relational Operator3/1
  CoEng_stShutOffPath/1 -> Bitwise Operator1/1
  Switch/1 -> EngBrk_stNTCModeCurr/1  "EngBrk_stNTCModeCurr"
  Constant4/1 -> Switch/1
  Constant3/1 -> Switch/3
  Logical Operator2/1 -> Switch/2, Logical Operator6/1
  Logical Operator1/1 -> Logical Operator2/1
  Logical Operator/1 -> Logical Operator2/2
  DSM_bEngBrkPSErr/1 -> Logical Operator1/1
  Relational Operator2/1 -> Logical Operator/2
  Relational Operator1/1 -> Logical Operator/1
  Constant2/1 -> Relational Operator2/2
  EngBrk_rExhFlpCurr/1 -> Relational Operator2/1
  EngBrk_rECRCurr/1 -> Relational Operator1/1

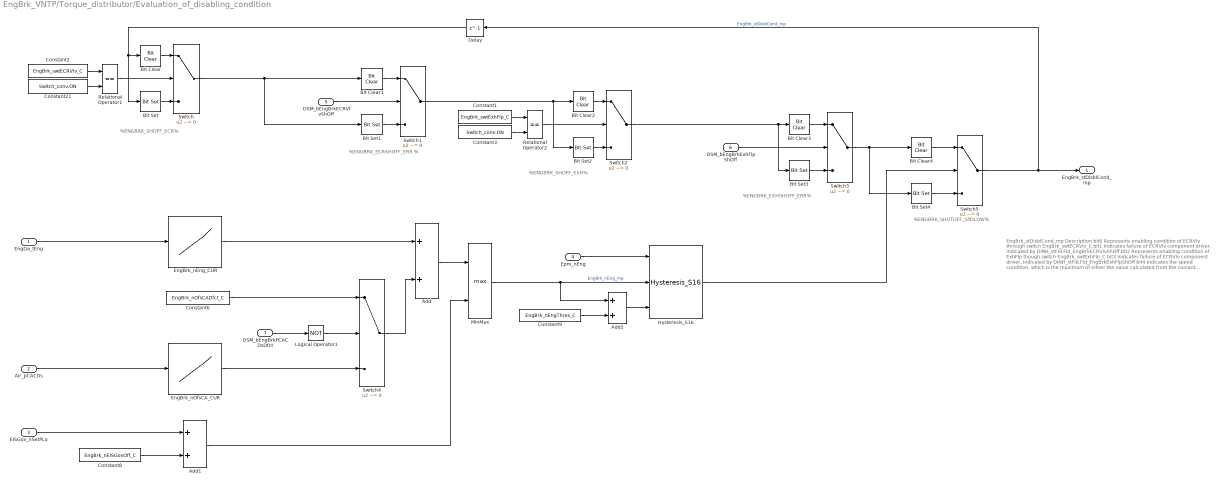
== system EngBrk_VNTP/Torque_distributor/Evaluation_of_disabling_condition ==
  note: EngBrk_stDisblCond_mp
      | Description
      |
      | bit0
      | Represents enabling condition of ECRVlv through switch EngBrk_swtECRVlv_C
      |
      | bit1
      | Indicates failure of ECRVlv component driver, indicated by DINH_stFId.FId_EngBrkECRVlvShOff
      |
      | bit2
      | Represents enabling condition of ExhFlp though switch EngBrk_swtExhFlp_C
      |
      | bit3
      | Indicates failure of ECRVlv component driver, indicated by DINH_stFId.FId_EngBrkExhFlpShOff
      |
      | bit4
      | Indicates the speed condition, which is the maximum of either the value calculated from the coolant
      | temperature and the boost pressure or EISGov Set point
  note: %ENGBRK_SHOFF_ECR%
  note: %ENGBRK_ECRSHOFF_ERR %
  note: %ENGBRK_SHOFF_EXH%
  note: %ENGBRK_EXHSHOFF_ERR%
  note: %ENGBRK_SHUTOFF_SPDLOW%
  EngDa_tEng : Inport
  Air_pCACDs : Inport  Port=2
  EISGov_nSetPLo : Inport  Port=3
  Epm_nEng : Inport  Port=4
  DSM_bEngBrkECRVlvShOff : Inport  Description=state of FId_EngBrkECRVlvShOff  Port=5  OutMin=0  OutMax=1  OutDataTypeStr=boolean
  DSM_bEngBrkExhFlpShOff : Inport  Description=state of FId_EngBrkExhFlpShOff  Port=6  OutMin=0  OutMax=1  OutDataTypeStr=boolean
  DSM_bEngBrkPCACDsDfct : Inport  Description=state of FId_EngBrkPCACDsDfct  Port=7  OutMin=0  OutMax=1  OutDataTypeStr=boolean
  Add : Sum  SaturateOnIntegerOverflow=on  InputSameDT=on
  Add1 : Sum  SaturateOnIntegerOverflow=on  InputSameDT=on
  Add2 : Sum  SaturateOnIntegerOverflow=on  InputSameDT=on
  Bit Clear : simulink/Logic and Bit Operations/Bit Clear  iBit=0
  Bit Clear1 : simulink/Logic and Bit Operations/Bit Clear  iBit=1
  Bit Clear2 : simulink/Logic and Bit Operations/Bit Clear  iBit=2
  Bit Clear3 : simulink/Logic and Bit Operations/Bit Clear  iBit=3
  Bit Clear4 : simulink/Logic and Bit Operations/Bit Clear  iBit=4
  Bit Set : simulink/Logic and Bit Operations/Bit Set  iBit=0
  Bit Set1 : simulink/Logic and Bit Operations/Bit Set  iBit=1
  Bit Set2 : simulink/Logic and Bit Operations/Bit Set  iBit=2
  Bit Set3 : simulink/Logic and Bit Operations/Bit Set  iBit=3
  Bit Set4 : simulink/Logic and Bit Operations/Bit Set  iBit=4
  Constant1 : Constant  Value=EngBrk_swtExhFlp_C
  Constant2 : Constant  Value=EngBrk_swtECRVlv_C
  Constant21 : Constant  Value=Switch_conv.ON  OutDataTypeStr=Inherit: Inherit via back propagation
  Constant3 : Constant  Value=Switch_conv.ON  OutDataTypeStr=Inherit: Inherit via back propagation
  Constant6 : Constant  Value=EngBrk_nOfsCADfct_C
  Constant8 : Constant  Value=EngBrk_nEISGovOff_C
  Constant9 : Constant  Value=EngBrk_nEngThres_C
  Delay : Delay  DelayLength=1  InitialCondition=0
  EngBrk_nEng_CUR : Lookup_n-D  NumberOfTableDimensions=1  BreakpointsForDimension1=EngBrk_nEng_CURX  BreakpointsForDimension2=HPUn_etaPmp_MAPY  IndexSearchMethod=Linear search  BeginIndexSearchUsingPreviousIndexResult=on  Table=EngBrk_nEng_CUR  ExtrapMethod=Clip  UseLastTableValue=on  InternalRulePriority=Speed  OutDataTypeStr=Inherit: Inherit via back propagation  SaturateOnIntegerOverflow=on
  EngBrk_nOfsCA_CUR : Lookup_n-D  NumberOfTableDimensions=1  BreakpointsForDimension1=EngBrk_nOfsCA_CURX  BreakpointsForDimension2=HPUn_etaPmp_MAPY  IndexSearchMethod=Linear search  BeginIndexSearchUsingPreviousIndexResult=on  Table=EngBrk_nOfsCA_CUR  ExtrapMethod=Clip  UseLastTableValue=on  InternalRulePriority=Speed  OutDataTypeStr=Inherit: Inherit via back propagation  SaturateOnIntegerOverflow=on
  Hysteresis_S16 : CXLib/Hysteresis_S16
  Logical Operator1 : Logic  Operator=NOT  AllPortsSameDT=off  OutDataTypeStr=boolean
  MinMax : MinMax  Function=max  Inputs=2  SaturateOnIntegerOverflow=on  InputSameDT=on
  Relational Operator1 : RelationalOperator  Operator===  OutDataTypeStr=boolean  RndMeth=Simplest  InputSameDT=on
  Relational Operator2 : RelationalOperator  Operator===  OutDataTypeStr=boolean  RndMeth=Simplest  InputSameDT=on
  Switch{,1..4} (5 alike) : Switch  Criteria=u2 ~= 0  SaturateOnIntegerOverflow=on  InputSameDT=on
  Switch5 : Switch  Criteria=u2 ~= 0  InputSameDT=on
  EngBrk_stDisblCond_mp : Outport
  wires:
  Delay/1 -> Bit Clear/1, Bit Set/1
  Switch5/1 -> Delay/1, EngBrk_stDisblCond_mp/1  "EngBrk_stDisblCond_mp"
  Switch3/1 -> Bit Clear4/1, Bit Set4/1
  Bit Clear4/1 -> Switch5/1
  Bit Set4/1 -> Switch5/3
  Hysteresis_S16/1 -> Switch5/2
  Constant9/1 -> Add2/2
  Add2/1 -> Hysteresis_S16/3
  MinMax/1 -> Add2/1, Hysteresis_S16/2  "EngBrk_nEng_mp"
  Epm_nEng/1 -> Hysteresis_S16/1
  Add1/1 -> MinMax/2
  Constant8/1 -> Add1/2
  EISGov_nSetPLo/1 -> Add1/1
  Add/1 -> MinMax/1
  EngBrk_nEng_CUR/1 -> Add/1
  Switch4/1 -> Add/2
  Constant6/1 -> Switch4/1
  Logical Operator1/1 -> Switch4/2
  DSM_bEngBrkPCACDsDfct/1 -> Logical Operator1/1
  EngBrk_nOfsCA_CUR/1 -> Switch4/3
  Air_pCACDs/1 -> EngBrk_nOfsCA_CUR/1
  EngDa_tEng/1 -> EngBrk_nEng_CUR/1
  Switch2/1 -> Bit Clear3/1, Bit Set3/1
  Bit Set3/1 -> Switch3/3
  Bit Clear3/1 -> Switch3/1
  DSM_bEngBrkExhFlpShOff/1 -> Switch3/2
  Switch1/1 -> Bit Clear2/1, Bit Set2/1
  Bit Clear2/1 -> Switch2/1
  Bit Set2/1 -> Switch2/3
  Relational Operator2/1 -> Switch2/2
  Constant3/1 -> Relational Operator2/2
  Constant1/1 -> Relational Operator2/1
  Switch/1 -> Bit Clear1/1, Bit Set1/1
  Bit Set1/1 -> Switch1/3
  Bit Clear1/1 -> Switch1/1
  DSM_bEngBrkECRVlvShOff/1 -> Switch1/2
  Bit Clear/1 -> Switch/1
  Bit Set/1 -> Switch/3
  Relational Operator1/1 -> Switch/2
  Constant21/1 -> Relational Operator1/2
  Constant2/1 -> Relational Operator1/1

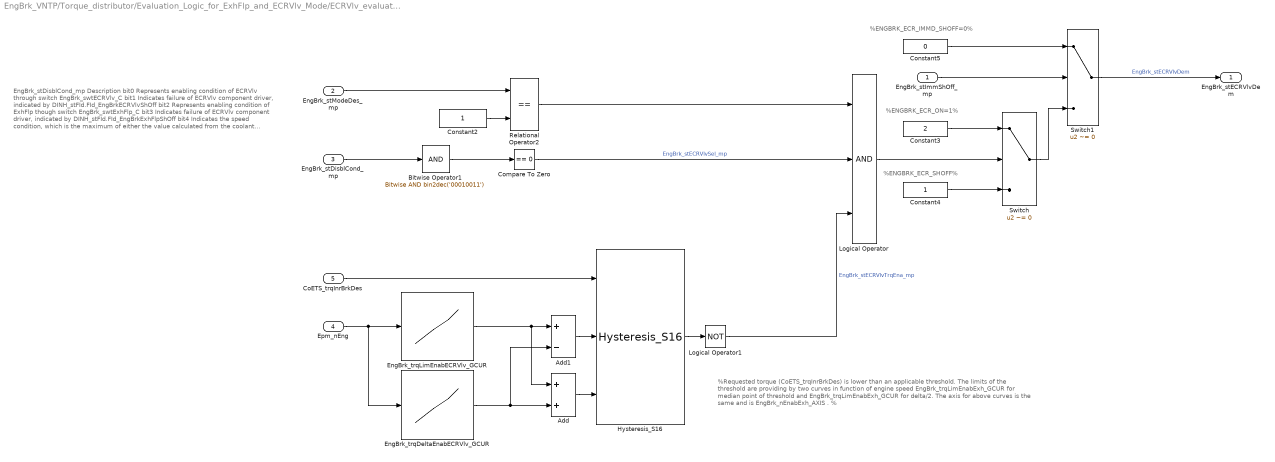
== system EngBrk_VNTP/Torque_distributor/Evaluation_Logic_for_ExhFlp_and_ECRVlv_Mode/ECRVlv_evaluation ==
  note: EngBrk_stDisblCond_mp
      | Description
      |
      | bit0
      | Represents enabling condition of ECRVlv through switch EngBrk_swtECRVlv_C
      |
      | bit1
      | Indicates failure of ECRVlv component driver, indicated by DINH_stFId.FId_EngBrkECRVlvShOff
      |
      | bit2
      | Represents enabling condition of ExhFlp though switch EngBrk_swtExhFlp_C
      |
      | bit3
      | Indicates failure of ECRVlv component driver, indicated by DINH_stFId.FId_EngBrkExhFlpShOff
      |
      | bit4
      | Indicates the speed condition, which is the maximum of either the value calculated from the coolant
      | temperature and the boost pressure or EISGov Set point
  note: %ENGBRK_ECR_IMMD_SHOFF=0%
  note: %ENGBRK_ECR_ON=1%
  note: %ENGBRK_ECR_SHOFF%
  note: %Requested torque (CoETS_trqInrBrkDes) is lower than an applicable threshold. The limits of the threshold are providing by two curves in
      | function of engine speed EngBrk_trqLimEnabExh_GCUR for median point of threshold and EngBrk_trqLimEnabExh_GCUR for delta/2.
      | The axis for above curves is the same and is EngBrk_nEnabExh_AXIS . %
  EngBrk_stImmShOff_mp : Inport
  EngBrk_stModeDes_mp : Inport  Port=2
  EngBrk_stDisblCond_mp : Inport  Port=3
  Epm_nEng : Inport  Port=4
  CoETS_trqInrBrkDes : Inport  Port=5
  Add : Sum  InputSameDT=on
  Add1 : Sum  Inputs=+-  OutDataTypeStr=Inherit: Inherit via back propagation  InputSameDT=on
  Bitwise Operator1 : simulink/Logic and Bit Operations/Bitwise Operator  logicop=AND  UseBitMask=on  BitMask=bin2dec('00010011')  BitMaskRealWorld=Stored Integer
  Compare To Zero : simulink/Logic and Bit Operations/Compare To Zero  relop===  OutDataTypeStr=boolean
  Constant2 : Constant  OutDataTypeStr=Inherit: Inherit via back propagation
  Constant3 : Constant  Value=2  OutDataTypeStr=Inherit: Inherit via back propagation
  Constant4 : Constant  OutDataTypeStr=Inherit: Inherit via back propagation
  Constant5 : Constant  Value=0  OutDataTypeStr=Inherit: Inherit via back propagation
  EngBrk_trqDeltaEnabECRVlv_GCUR : Lookup_n-D  NumberOfTableDimensions=1  BreakpointsForDimension1=EngBrk_trqDeltaEnabECRVlv_GCURX  BreakpointsForDimension2=HPUn_etaPmp_MAPY  IndexSearchMethod=Linear search  BeginIndexSearchUsingPreviousIndexResult=on  Table=EngBrk_trqDeltaEnabECRVlv_GCUR  ExtrapMethod=Clip  UseLastTableValue=on  InternalRulePriority=Speed  OutDataTypeStr=Inherit: Inherit via back propagation  SaturateOnIntegerOverflow=on
  EngBrk_trqLimEnabECRVlv_GCUR : Lookup_n-D  NumberOfTableDimensions=1  BreakpointsForDimension1=EngBrk_trqLimEnabECRVlv_GCURX  BreakpointsForDimension2=HPUn_etaPmp_MAPY  IndexSearchMethod=Linear search  BeginIndexSearchUsingPreviousIndexResult=on  Table=EngBrk_trqLimEnabECRVlv_GCUR  ExtrapMethod=Clip  UseLastTableValue=on  InternalRulePriority=Speed  OutDataTypeStr=Inherit: Inherit via back propagation  SaturateOnIntegerOverflow=on
  Hysteresis_S16 : CXLib/Hysteresis_S16
  Logical Operator : Logic  Inputs=3  OutDataTypeStr=boolean
  Logical Operator1 : Logic  Operator=NOT  AllPortsSameDT=off  OutDataTypeStr=boolean
  Relational Operator2 : RelationalOperator  Operator===  OutDataTypeStr=boolean  RndMeth=Simplest  InputSameDT=on
  Switch : Switch  Criteria=u2 ~= 0  SaturateOnIntegerOverflow=on  InputSameDT=on
  Switch1 : Switch  Criteria=u2 ~= 0  SaturateOnIntegerOverflow=on  InputSameDT=on
  EngBrk_stECRVlvDem : Outport
  wires:
  Logical Operator1/1 -> Logical Operator/3  "EngBrk_stECRVlvTrqEna_mp"
  Switch1/1 -> EngBrk_stECRVlvDem/1  "EngBrk_stECRVlvDem"
  Constant5/1 -> Switch1/1
  EngBrk_stImmShOff_mp/1 -> Switch1/2
  Switch/1 -> Switch1/3
  Constant4/1 -> Switch/3
  Constant3/1 -> Switch/1
  Logical Operator/1 -> Switch/2
  Relational Operator2/1 -> Logical Operator/1
  Constant2/1 -> Relational Operator2/2
  EngBrk_stModeDes_mp/1 -> Relational Operator2/1
  Compare To Zero/1 -> Logical Operator/2  "EngBrk_stECRVlvSel_mp"
  Hysteresis_S16/1 -> Logical Operator1/1
  Bitwise Operator1/1 -> Compare To Zero/1
  EngBrk_stDisblCond_mp/1 -> Bitwise Operator1/1
  Add/1 -> Hysteresis_S16/3
  EngBrk_trqDeltaEnabECRVlv_GCUR/1 -> Add/2, Add1/2
  EngBrk_trqLimEnabECRVlv_GCUR/1 -> Add1/1, Add/1
  Add1/1 -> Hysteresis_S16/2
  CoETS_trqInrBrkDes/1 -> Hysteresis_S16/1
  Epm_nEng/1 -> EngBrk_trqLimEnabECRVlv_GCUR/1, EngBrk_trqDeltaEnabECRVlv_GCUR/1

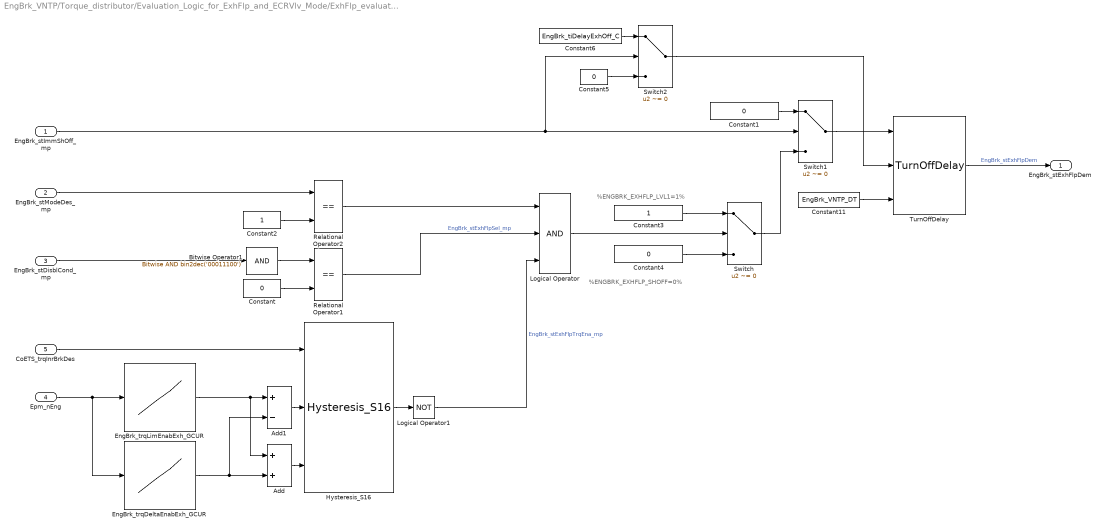
== system EngBrk_VNTP/Torque_distributor/Evaluation_Logic_for_ExhFlp_and_ECRVlv_Mode/ExhFlp_evaluation ==
  note: %ENGBRK_EXHFLP_SHOFF=0%
  note: %ENGBRK_EXHFLP_LVL1=1%
  EngBrk_stImmShOff_mp : Inport
  EngBrk_stModeDes_mp : Inport  Port=2
  EngBrk_stDisblCond_mp : Inport  Port=3
  Epm_nEng : Inport  Port=4
  CoETS_trqInrBrkDes : Inport  Port=5
  Add : Sum  InputSameDT=on
  Add1 : Sum  Inputs=+-  OutDataTypeStr=Inherit: Inherit via back propagation  InputSameDT=on
  Bitwise Operator1 : simulink/Logic and Bit Operations/Bitwise Operator  logicop=AND  UseBitMask=on  BitMask=bin2dec('00011100')  BitMaskRealWorld=Stored Integer
  Constant : Constant  Value=0  OutDataTypeStr=Inherit: Inherit via back propagation
  Constant1 : Constant  Value=0  OutDataTypeStr=boolean
  Constant11 : Constant  Value=EngBrk_VNTP_DT  OutDataTypeStr=Inherit: Inherit via back propagation
  Constant2 : Constant  OutDataTypeStr=Inherit: Inherit via back propagation
  Constant3 : Constant  OutDataTypeStr=boolean
  Constant4 : Constant  Value=0  OutDataTypeStr=boolean
  Constant5 : Constant  Value=0  OutDataTypeStr=Inherit: Inherit via back propagation
  Constant6 : Constant  Value=EngBrk_tiDelayExhOff_C
  EngBrk_trqDeltaEnabExh_GCUR : Lookup_n-D  NumberOfTableDimensions=1  BreakpointsForDimension1=EngBrk_trqDeltaEnabExh_GCURX  BreakpointsForDimension2=HPUn_etaPmp_MAPY  IndexSearchMethod=Linear search  BeginIndexSearchUsingPreviousIndexResult=on  Table=EngBrk_trqDeltaEnabExh_GCUR  ExtrapMethod=Clip  UseLastTableValue=on  InternalRulePriority=Speed  OutDataTypeStr=Inherit: Inherit via back propagation  SaturateOnIntegerOverflow=on
  EngBrk_trqLimEnabExh_GCUR : Lookup_n-D  NumberOfTableDimensions=1  BreakpointsForDimension1=EngBrk_trqLimEnabExh_GCURX  BreakpointsForDimension2=HPUn_etaPmp_MAPY  IndexSearchMethod=Linear search  BeginIndexSearchUsingPreviousIndexResult=on  Table=EngBrk_trqLimEnabExh_GCUR  ExtrapMethod=Clip  UseLastTableValue=on  InternalRulePriority=Speed  OutDataTypeStr=Inherit: Inherit via back propagation  SaturateOnIntegerOverflow=on
  Hysteresis_S16 : CXLib/Hysteresis_S16
  Logical Operator : Logic  Inputs=3  OutDataTypeStr=boolean
  Logical Operator1 : Logic  Operator=NOT  AllPortsSameDT=off  OutDataTypeStr=boolean
  Relational Operator1 : RelationalOperator  Operator===  OutDataTypeStr=boolean  RndMeth=Nearest  InputSameDT=on
  Relational Operator2 : RelationalOperator  Operator===  OutDataTypeStr=boolean  RndMeth=Simplest  InputSameDT=on
  Switch : Switch  Criteria=u2 ~= 0  SaturateOnIntegerOverflow=on  InputSameDT=on
  Switch1 : Switch  Criteria=u2 ~= 0  SaturateOnIntegerOverflow=on  InputSameDT=on
  Switch2 : Switch  Criteria=u2 ~= 0  SaturateOnIntegerOverflow=on  InputSameDT=on
  TurnOffDelay : CXLib/TurnOffDelay
  EngBrk_stExhFlpDem : Outport
  wires:
  Logical Operator1/1 -> Logical Operator/3  "EngBrk_stExhFlpTrqEna_mp"
  Constant1/1 -> Switch1/1
  Constant11/1 -> TurnOffDelay/3
  Switch2/1 -> TurnOffDelay/2
  Constant6/1 -> Switch2/1
  Constant5/1 -> Switch2/3
  TurnOffDelay/1 -> EngBrk_stExhFlpDem/1  "EngBrk_stExhFlpDem"
  Switch1/1 -> TurnOffDelay/1
  EngBrk_stImmShOff_mp/1 -> Switch1/2, Switch2/2
  Switch/1 -> Switch1/3
  Constant4/1 -> Switch/3
  Constant3/1 -> Switch/1
  Logical Operator/1 -> Switch/2
  Relational Operator2/1 -> Logical Operator/1
  Constant2/1 -> Relational Operator2/2
  EngBrk_stModeDes_mp/1 -> Relational Operator2/1
  Relational Operator1/1 -> Logical Operator/2  "EngBrk_stExhFlpSel_mp"
  Hysteresis_S16/1 -> Logical Operator1/1
  Constant/1 -> Relational Operator1/2
  EngBrk_stDisblCond_mp/1 -> Bitwise Operator1/1
  Add/1 -> Hysteresis_S16/3
  EngBrk_trqDeltaEnabExh_GCUR/1 -> Add/2, Add1/2
  EngBrk_trqLimEnabExh_GCUR/1 -> Add1/1, Add/1
  Add1/1 -> Hysteresis_S16/2
  CoETS_trqInrBrkDes/1 -> Hysteresis_S16/1
  Epm_nEng/1 -> EngBrk_trqLimEnabExh_GCUR/1, EngBrk_trqDeltaEnabExh_GCUR/1
  Bitwise Operator1/1 -> Relational Operator1/1
